simulink model "em_track_sim"  (R2025a)
settings: Solver=FixedStepDiscrete  StartTime=0.0  StopTime=P.stopTime  FixedStep=P.dt  RelTol=1e-3
InitFcn:
  | em_ensure_init;
values from neighbouring files (symbols this model uses):
  P = params()    [init.m]
  TD = struct('name', trk.name, 'segs', {trk.segs}, 'closed', trk.closed,      'wires', wires, 'mids', mids, 'dls', dls, 'path', path, 'length', path.len)    [build_track_data.m]    (also in init.m = build_track_data(P.trackName, P))
libraries: simulink x1
settings Model: Creator=Li  LastModifiedBy=Li

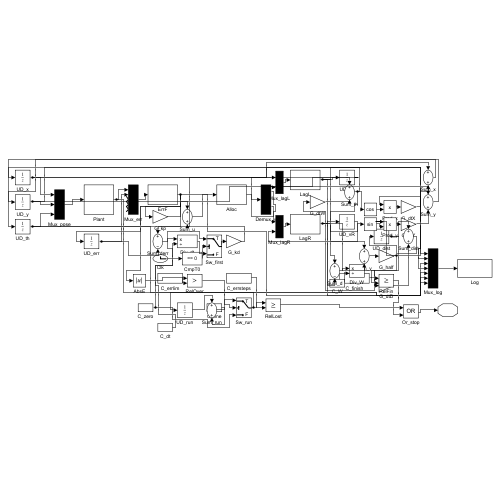
[thumbnail: Simulink's stored preview of the top-level diagram]
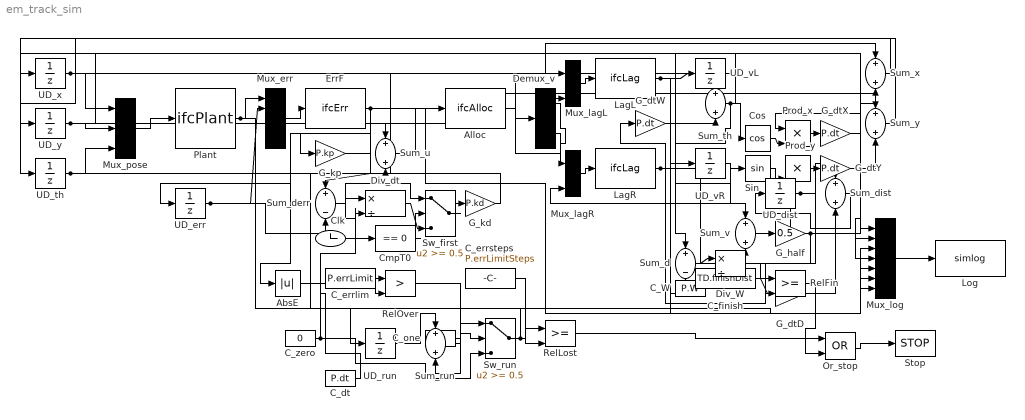
== system em_track_sim ==
  AbsE : Abs  SaturateOnIntegerOverflow=off
  Alloc : MATLABFcn  MATLABFcn=ifcAlloc  OutputDimensions=2
  C_W : Constant  Value=P.W
  C_dt : Constant  Value=P.dt
  C_errlim : Constant  Value=P.errLimit
  C_errsteps : Constant  Value=P.errLimitSteps
  C_finish : Constant  Value=TD.finishDist
  C_one : Constant
  C_zero : Constant  Value=0
  Clk : Clock
  CmpT0 : simulink/Logic and Bit Operations/Compare To Constant  relop===  const=0  OutDataTypeStr=boolean
  Cos : Trigonometry  Operator=cos
  Demux_v : Demux  Outputs=2
  Div_W : Product  Inputs=*/
  Div_dt : Product  Inputs=*/
  ErrF : MATLABFcn  MATLABFcn=ifcErr  OutputDimensions=1
  G_dtD : Gain  Gain=P.dt
  G_dtW : Gain  Gain=P.dt
  G_dtX : Gain  Gain=P.dt
  G_dtY : Gain  Gain=P.dt
  G_half : Gain  Gain=0.5
  G_kd : Gain  Gain=P.kd
  G_kp : Gain  Gain=P.kp
  LagL : MATLABFcn  MATLABFcn=ifcLag  OutputDimensions=1
  LagR : MATLABFcn  MATLABFcn=ifcLag  OutputDimensions=1
  Log : ToWorkspace  VariableName=simlog  SaveFormat=Structure With Time  SampleTime=-1
  Mux_err : Mux  Inputs=5
  Mux_lagL : Mux  Inputs=2
  Mux_lagR : Mux  Inputs=2
  Mux_log : Mux  Inputs=7
  Mux_pose : Mux  Inputs=3
  Or_stop : Logic  Operator=OR  AllPortsSameDT=off  OutDataTypeStr=boolean
  Plant : MATLABFcn  MATLABFcn=ifcPlant  OutputDimensions=4
  Prod_x : Product
  Prod_y : Product
  RelFin : RelationalOperator  OutDataTypeStr=boolean  RndMeth=Simplest  InputSameDT=off
  RelLost : RelationalOperator  OutDataTypeStr=boolean  RndMeth=Simplest  InputSameDT=off
  RelOver : RelationalOperator  Operator=>  OutDataTypeStr=boolean  RndMeth=Simplest  InputSameDT=off
  Sin : Trigonometry
  Stop : Stop
  Sum_d : Sum  Inputs=+-
  Sum_derr : Sum  Inputs=+-
  Sum_dist : Sum
  Sum_run : Sum
  Sum_th : Sum
  Sum_u : Sum
  Sum_v : Sum
  Sum_x : Sum
  Sum_y : Sum
  Sw_first : Switch  Threshold=0.5  SaturateOnIntegerOverflow=off  InputSameDT=off
  Sw_run : Switch  Threshold=0.5  SaturateOnIntegerOverflow=off  InputSameDT=off
  UD_dist : UnitDelay  SampleTime=-1  HasFrameUpgradeWarning=on
  UD_err : UnitDelay  SampleTime=-1  HasFrameUpgradeWarning=on
  UD_run : UnitDelay  SampleTime=-1  HasFrameUpgradeWarning=on
  UD_th : UnitDelay  InitialCondition=TD.theta0  SampleTime=-1  HasFrameUpgradeWarning=on
  UD_vL : UnitDelay  InitialCondition=P.vBase  SampleTime=-1  HasFrameUpgradeWarning=on
  UD_vR : UnitDelay  InitialCondition=P.vBase  SampleTime=-1  HasFrameUpgradeWarning=on
  UD_x : UnitDelay  InitialCondition=TD.x0  SampleTime=-1  HasFrameUpgradeWarning=on
  UD_y : UnitDelay  InitialCondition=TD.y0  SampleTime=-1  HasFrameUpgradeWarning=on
  wires:
  UD_x/1 -> Mux_pose/1, Sum_x/1, Mux_log/1
  UD_y/1 -> Mux_pose/2, Sum_y/1, Mux_log/2
  UD_th/1 -> Mux_pose/3, Sum_th/1, Mux_log/3
  Mux_pose/1 -> Plant/1
  Plant/1 -> Mux_err/1, Mux_log/7
  UD_err/1 -> Mux_err/2, Sum_derr/2
  Mux_err/1 -> ErrF/1
  ErrF/1 -> Sum_derr/1, G_kp/1, UD_err/1, AbsE/1, Mux_log/6
  Sum_derr/1 -> Div_dt/1
  C_dt/1 -> Div_dt/2
  Div_dt/1 -> Sw_first/3
  C_zero/1 -> Sw_first/1, Sw_run/3
  Clk/1 -> CmpT0/1
  CmpT0/1 -> Sw_first/2
  Sw_first/1 -> G_kd/1
  G_kp/1 -> Sum_u/1
  G_kd/1 -> Sum_u/2
  Sum_u/1 -> Alloc/1
  Alloc/1 -> Demux_v/1
  Demux_v/1 -> Mux_lagL/1
  UD_vL/1 -> Mux_lagL/2
  Mux_lagL/1 -> LagL/1
  Demux_v/2 -> Mux_lagR/1
  UD_vR/1 -> Mux_lagR/2
  Mux_lagR/1 -> LagR/1
  LagL/1 -> UD_vL/1, Sum_v/1, Sum_d/2, Mux_log/4
  LagR/1 -> UD_vR/1, Sum_v/2, Sum_d/1, Mux_log/5
  Sum_v/1 -> G_half/1
  Sum_d/1 -> Div_W/1
  C_W/1 -> Div_W/2
  Div_W/1 -> G_dtW/1
  G_dtW/1 -> Sum_th/2
  Sum_th/1 -> UD_th/1, Cos/1, Sin/1
  G_half/1 -> Prod_x/1, Prod_y/1, G_dtD/1
  Cos/1 -> Prod_x/2
  Sin/1 -> Prod_y/2
  Prod_x/1 -> G_dtX/1
  Prod_y/1 -> G_dtY/1
  G_dtX/1 -> Sum_x/2
  Sum_x/1 -> UD_x/1
  G_dtY/1 -> Sum_y/2
  Sum_y/1 -> UD_y/1
  UD_dist/1 -> Sum_dist/1, RelFin/1
  G_dtD/1 -> Sum_dist/2
  Sum_dist/1 -> UD_dist/1
  AbsE/1 -> RelOver/1
  C_errlim/1 -> RelOver/2
  UD_run/1 -> Sum_run/1
  C_one/1 -> Sum_run/2
  Sum_run/1 -> Sw_run/1
  RelOver/1 -> Sw_run/2
  Sw_run/1 -> UD_run/1, RelLost/1
  C_errsteps/1 -> RelLost/2
  C_finish/1 -> RelFin/2
  RelLost/1 -> Or_stop/1
  RelFin/1 -> Or_stop/2
  Or_stop/1 -> Stop/1
  Mux_log/1 -> Log/1
